simulink model "demo_simulink_2022b"  (R2023a)
settings: Solver=ode23  StartTime=0.0  StopTime=20  RelTol=1e-3
undefined symbols (not defined in the file): alpha, ALPHA, BETA, GAMMA, k, m, V, v_0, x_0
libraries: simulink x4
settings Model: Creator=Артём  LastModifiedBy=nikit
settings SolverCC: ZeroCrossAlgorithm=Adaptive
settings DebuggingCC: IgnoredZcDiagnostic=none

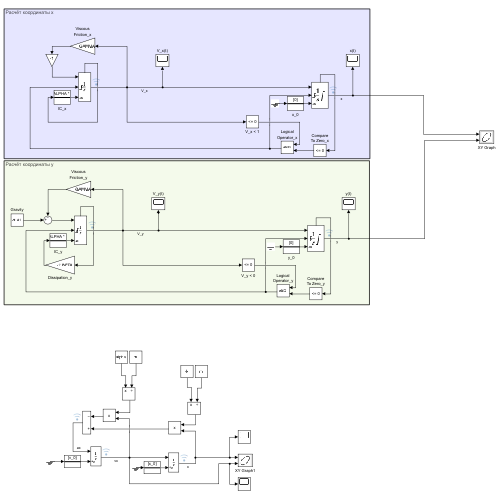
[thumbnail: Simulink's stored preview of the top-level diagram]
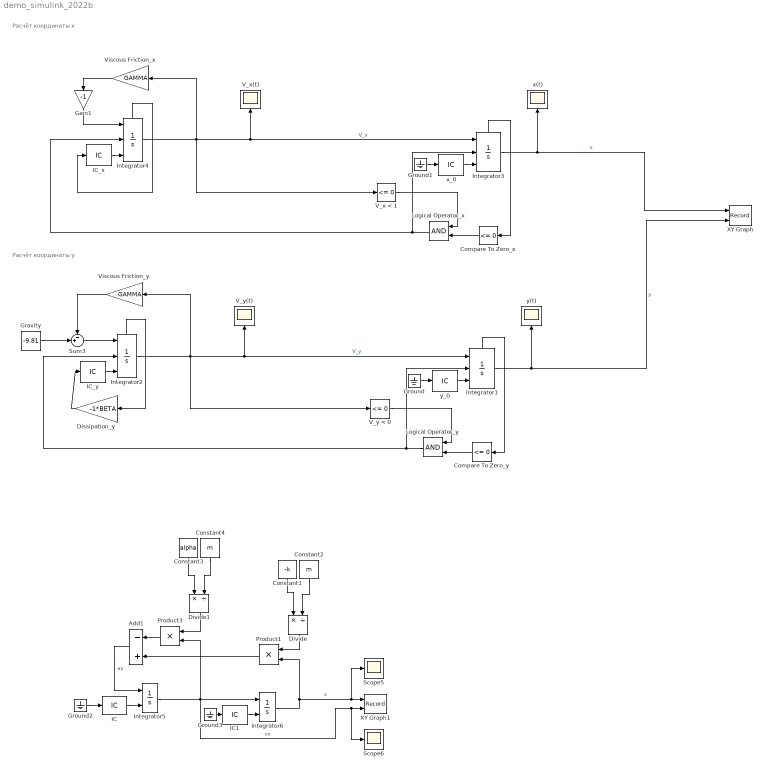
== system demo_simulink_2022b ==
  note: Расчёт координаты y
  note: Расчёт координаты x
  Add1 : Sum  Inputs=-+
  Compare To Zero_x : simulink/Logic and Bit Operations/Compare To Zero  relop=<=  OutDataTypeStr=boolean
  Compare To Zero_y : simulink/Logic and Bit Operations/Compare To Zero  relop=<=  OutDataTypeStr=boolean
  Constant1 : Constant  Value=-k
  Constant2 : Constant  Value=m
  Constant3 : Constant  Value=alpha
  Constant4 : Constant  Value=m
  Dissipation_y : Gain  Gain=-1*BETA
  Divide : Product  Inputs=*/
  Divide1 : Product  Inputs=*/
  Gain1 : Gain  Gain=-1
  Gravity : Constant  Value=-9.81
  Ground{,1..3} (4 alike) : Ground
  IC : InitialCondition  Value=v_0
  IC1 : InitialCondition  Value=x_0
  IC_x : InitialCondition  Value=V * cos(ALPHA * pi / 180)
  IC_y : InitialCondition  Value=V * sin(ALPHA * pi / 180)
  Integrator1 : Integrator  ExternalReset=rising  InitialConditionSource=external  LimitOutput=on  LowerSaturationLimit=0  ShowStatePort=on
  Integrator2 : Integrator  ExternalReset=rising  InitialConditionSource=external  ShowStatePort=on
  Integrator3 : Integrator  ExternalReset=rising  InitialConditionSource=external  LimitOutput=on  LowerSaturationLimit=0  ShowStatePort=on
  Integrator4 : Integrator  ExternalReset=rising  InitialConditionSource=external  ShowStatePort=on
  Integrator5 : Integrator  InitialConditionSource=external
  Integrator6 : Integrator  InitialConditionSource=external
  Logical Operator_x : Logic  AllPortsSameDT=off  OutDataTypeStr=boolean
  Logical Operator_y : Logic  AllPortsSameDT=off  OutDataTypeStr=boolean
  Product1 : Product
  Product3 : Product
  Scope5 : Scope
  Scope6 : Scope
  Sum3 : Sum  Inputs=-+|
  V_x < 1 : simulink/Logic and Bit Operations/Compare To Zero  relop=<=  OutDataTypeStr=boolean
  V_x(t) : Scope
  V_y < 0 : simulink/Logic and Bit Operations/Compare To Zero  relop=<=  OutDataTypeStr=boolean
  V_y(t) : Scope
  Viscous Friction_x : Gain  Gain=GAMMA
  Viscous Friction_y : Gain  Gain=GAMMA
  XY Graph : Record  FileSettingsInternal="{\"entries\":[{\"content\":{\"excelSettings\":{\"content\":{},\"type\":\"Streamout.ExcelSettings\"}},\"type\":\"Streamout.FileSettingStorage\",\"uuid\":\"\"}],\"packageUris\":[\"http:\\/\\/schema.mathworks.com\\/mf0\\/streamout_blocks\\/R2020a\"],\"version\":\"1.0\"}"  Layout=[1 1]  SignalsInternal="{\"entries\":[{\"content\":{\"signals\":[{\"content\":{\"blockPath\":[],\"dimensions\":[1],\"domain\":\"\",\"lineColor\":\"#b746ff\",\"plots\":[1],\"port\":1,\"sid\":[\"\"],\"signalID\":718,\"signalName\":\"x\"},\"type\":\"RecordBlkView.Signal\",\"uuid\":\"\"},{\"content\":{\"blockPath\":[],\"dimensions\":[1],\"domain\":\"\",\"lineColor\":\"#64d413\",\"plots\":[1],\"port\":2,\"sid\":[\"\"],\"signalID\":722,\"signalName\":\"y\"},\"type\":\"RecordBlkView.Signal\",\"uuid\":\"\"}]},\"type\":\"RecordBlkView.InputSignals\",\"uuid\":\"\"}],\"packageUris\":[\"http:\\/\\/schema.mathworks.com\\/mf0\\/streamout_blocks\\/R2020a\"],\"version\":\"1.0\"}"  VisualizationBindings="{\"xyplotplugin\":{\"info\":[{\"series\":[{\"bindingParametersList\":[{\"parameter\":\"Y-Axis\",\"signalID\":722,\"signalName\":\"y\"},{\"parameter\":\"X-Axis\",\"signalID\":718,\"signalName\":\"x\"}],\"seriesID\":4296}],\"subplotID\":1}]}}"  CompatibilityTag=XY
  XY Graph1 : Record  FileSettingsInternal="{\"entries\":[{\"content\":{\"excelSettings\":{\"content\":{},\"type\":\"Streamout.ExcelSettings\"}},\"type\":\"Streamout.FileSettingStorage\",\"uuid\":\"\"}],\"packageUris\":[\"http:\\/\\/schema.mathworks.com\\/mf0\\/streamout_blocks\\/R2020a\"],\"version\":\"1.0\"}"  Layout=[1 1]  SignalsInternal="{\"entries\":[{\"content\":{\"signals\":[{\"content\":{\"blockPath\":[],\"dimensions\":[1],\"domain\":\"\",\"lineColor\":\"#a2142f\",\"plots\":[1],\"port\":1,\"sid\":[\"\"],\"signalID\":694,\"signalName\":\"x\"},\"type\":\"RecordBlkView.Signal\",\"uuid\":\"\"},{\"content\":{\"blockPath\":[],\"dimensions\":[1],\"domain\":\"\",\"lineColor\":\"#139fff\",\"plots\":[1],\"port\":2,\"sid\":[\"\"],\"signalID\":698,\"signalName\":\"vx\"},\"type\":\"RecordBlkView.Signal\",\"uuid\":\"\"}]},\"type\":\"RecordBlkView.InputSignals\",\"uuid\":\"\"}],\"packageUris\":[\"http:\\/\\/schema.mathworks.com\\/mf0\\/streamout_blocks\\/R2020a\"],\"version\":\"1.0\"}"  VisualizationBindings="{\"xyplotplugin\":{\"info\":[{\"series\":[{\"bindingParametersList\":[{\"parameter\":\"X-Axis\",\"signalID\":694,\"signalName\":\"x\"},{\"parameter\":\"Y-Axis\",\"signalID\":698,\"signalName\":\"vx\"}],\"seriesID\":60278}],\"subplotID\":1}]}}"  CompatibilityTag=XY
  x(t) : Scope
  x_0 : InitialCondition  Value=0
  y(t) : Scope
  y_0 : InitialCondition  Value=0
  wires:
  Integrator2/1 -> Viscous Friction_y/1, V_y < 0/1, V_y(t)/1, Integrator1/1  "V_y"
  Integrator1/1 -> XY Graph/2, y(t)/1  "y"
  IC_y/1 -> Integrator2/3
  Logical Operator_y/1 -> Integrator2/2, Integrator1/2
  y_0/1 -> Integrator1/3
  Dissipation_y/1 -> IC_y/1
  Gravity/1 -> Sum3/2
  Ground/1 -> y_0/1
  V_y < 0/1 -> Logical Operator_y/1
  Integrator2/State -> Dissipation_y/1
  Integrator1/State -> Compare To Zero_y/1
  Viscous Friction_y/1 -> Sum3/1
  Sum3/1 -> Integrator2/1
  Gain1/1 -> Integrator4/1
  x_0/1 -> Integrator3/3
  V_x < 1/1 -> Logical Operator_x/1
  Integrator3/State -> Compare To Zero_x/1
  Integrator3/1 -> XY Graph/1, x(t)/1  "x"
  Compare To Zero_x/1 -> Logical Operator_x/2
  Viscous Friction_x/1 -> Gain1/1
  Ground1/1 -> x_0/1
  IC_x/1 -> Integrator4/3
  Integrator4/State -> IC_x/1
  Logical Operator_x/1 -> Integrator4/2, Integrator3/2
  Integrator4/1 -> Viscous Friction_x/1, V_x < 1/1, V_x(t)/1, Integrator3/1  "V_x"
  Compare To Zero_y/1 -> Logical Operator_y/2
  Constant1/1 -> Divide/1
  Constant2/1 -> Divide/2
  Divide/1 -> Product1/1
  Integrator6/1 -> XY Graph1/1, Scope5/1, Product1/2  "x"
  Divide1/1 -> Product3/1
  Integrator5/1 -> Product3/2, XY Graph1/2, Scope6/1, Integrator6/1  "vx"
  Constant3/1 -> Divide1/1
  Constant4/1 -> Divide1/2
  Product3/1 -> Add1/1
  Product1/1 -> Add1/2
  Add1/1 -> Integrator5/1  "ax"
  IC/1 -> Integrator5/2
  Ground2/1 -> IC/1
  Ground3/1 -> IC1/1
  IC1/1 -> Integrator6/2
